simulink model "windtest"  (Simulink 8.0)
settings: Solver=ode45  StartTime=0.0  StopTime=300  RelTol=1e-3
libraries: wt_blockset_v3 x3
settings Model: Creator=Administrator  LastModifiedBy=Administrator

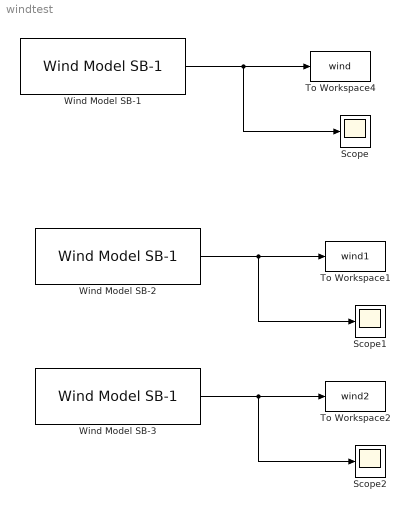
== system windtest ==
  Scope : Scope
  Scope1 : Scope
  Scope2 : Scope
      settings: SaveName=ScopeData2
  To Workspace1 : ToWorkspace  VariableName=wind1  SampleTime=-1
  To Workspace2 : ToWorkspace  VariableName=wind2  SampleTime=-1
  To Workspace4 : ToWorkspace  VariableName=wind  SampleTime=-1
  Wind Model SB-1 : wt_blockset_v3/Mechanical Components/Wind Model SB-1  D_rotor=72  v_mean=5  roughness=300  turb_int=12  T_sample=1
  Wind Model SB-2 : wt_blockset_v3/Mechanical Components/Wind Model SB-1  D_rotor=72  v_mean=10  roughness=300  turb_int=15  T_sample=1
  Wind Model SB-3 : wt_blockset_v3/Mechanical Components/Wind Model SB-1  D_rotor=72  v_mean=15  roughness=300  turb_int=12  T_sample=1
  wires:
  Wind Model SB-1/1 -> Scope/1, To Workspace4/1
  Wind Model SB-2/1 -> Scope1/1, To Workspace1/1
  Wind Model SB-3/1 -> Scope2/1, To Workspace2/1
